simulink model "Controller_Observer_Model"  (R2021b)
settings: Solver=FixedStepAuto  StartTime=0.0  StopTime=10.0  RelTol=1e-3  EnableMultiTasking=on
undefined symbols (not defined in the file): Ad, Bd, Cd, DiscIntNeverNeededParam, ki, Kp, L, Ts
settings Model: ExtModeTrigDuration=10  Creator=UTENTE  LastModifiedBy=UTENTE
settings OptimizationCC: EnhancedBackFolding=on  PassReuseOutputArgsAs=Individual arguments  ZeroExternalMemoryAtStartup=off  ZeroInternalMemoryAtStartup=off  MaxStackSize=64  OptimizeBlockOrder=speed  DifferentSizesBufferReuse=on  OptimizationCustomize=off  EfficientTunableParamExpr=on
settings DebuggingCC: ParameterTunabilityLossMsg=error
settings HardwareCC: ProdBitPerPointer=32  ProdBitPerSizeT=32  ProdBitPerPtrDiffT=32  ProdLargestAtomicInteger=Long  ProdLargestAtomicFloat=Double  ProdWordSize=32  ProdLongLongMode=on  ProdHWDeviceType=ARM Compatible->ARM Cortex
settings SFSimCC: MATLABDynamicMemAlloc=off
settings RTWCC: Description=Embedded Coder  SystemTargetFile=ert.tlc  HardwareBoard=STM32 Nucleo F401RE  TemplateMakefile=ert_default_tmf  Toolchain=GNU Tools for ARM Embedded Processors  PortableWordSizes=on
settings CodeAppCC: ForceParamTrailComments=on  IgnoreCustomStorageClasses=off  OperatorAnnotations=on  SimulinkDataObjDesc=on  SFDataObjDesc=on  InsertBlockDesc=on
settings ERTTargetCC: ExtModeTransport=3  ExtModeStaticAlloc=on  ExtModeStaticAllocSize=2000  ExtModeMexFile=ext_xcp  ExtModeIntrfLevel=Level2 - Open

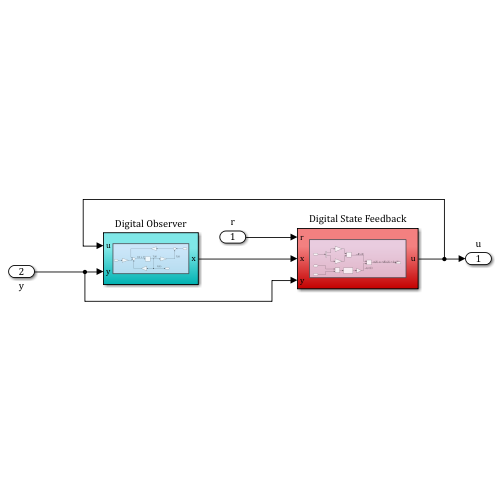
[thumbnail: Simulink's stored preview of the top-level diagram]
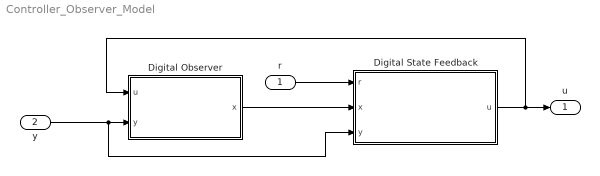
== system Controller_Observer_Model ==
  r : Inport
  y : Inport  Port=2
  Digital Observer : Subsystem
  Digital State Feedback : Subsystem
  u : Outport
  wires:
  r/1 -> Digital State Feedback/1(r)
  Digital State Feedback/1(u) -> Digital Observer/1(u), u/1
  Digital Observer/1(x) -> Digital State Feedback/2(x)
  y/1 -> Digital State Feedback/3(y), Digital Observer/2(y)

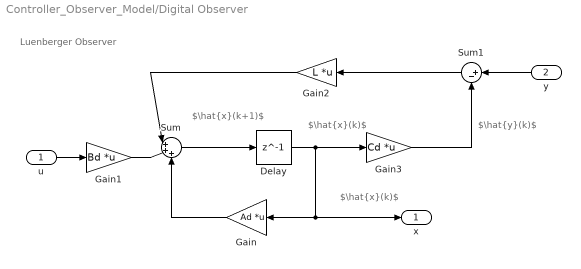
== system Controller_Observer_Model/Digital Observer ==
  note: $\hat{x}(k+1)$
  note: Luenberger Observer
  note: $\hat{x}(k)$
  note: $\hat{y}(k)$
  note: $\hat{x}(k)$
  u : Inport
  y : Inport  Port=2
  Delay : Delay  DelayLength=1  SampleTime=Ts
  Gain : Gain  Gain=Ad  Multiplication=Matrix(K*u)
  Gain1 : Gain  Gain=Bd  Multiplication=Matrix(K*u)
  Gain2 : Gain  Gain=L  Multiplication=Matrix(K*u)
  Gain3 : Gain  Gain=Cd  Multiplication=Matrix(K*u)
  Sum : Sum  Inputs=|+++
  Sum1 : Sum  Inputs=|+-
  x : Outport
  wires:
  u/1 -> Gain1/1
  Gain3/1 -> Sum1/2
  Delay/1 -> x/1, Gain/1, Gain3/1
  Gain1/1 -> Sum/2
  Gain2/1 -> Sum/1
  Sum/1 -> Delay/1
  Gain/1 -> Sum/3
  Sum1/1 -> Gain2/1
  y/1 -> Sum1/1

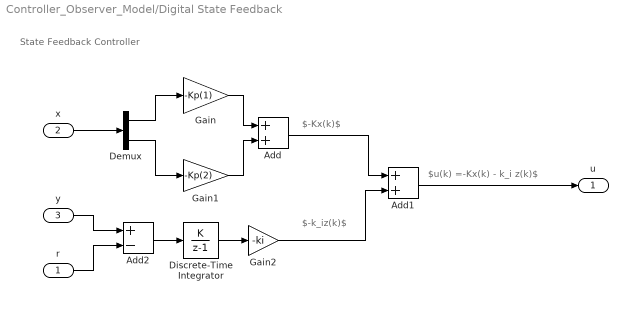
== system Controller_Observer_Model/Digital State Feedback ==
  note: $u(k) =-Kx(k) - k_i z(k)$
  note: $-k_iz(k)$
  note: $-Kx(k)$
  note: State Feedback Controller
  r : Inport
  x : Inport  Port=2
  y : Inport  Port=3
  Add : Sum
  Add1 : Sum
  Add2 : Sum  Inputs=+-
  Demux : Demux  Outputs=2
  Discrete-Time Integrator : DiscreteIntegrator  IntegratorMethod=Accumulation: Forward Euler  SampleTime=Ts  StateName='IntegralAction'  ICPrevOutput=DiscIntNeverNeededParam  ICPrevScaledInput=DiscIntNeverNeededParam
  Gain : Gain  Gain=-Kp(1)
  Gain1 : Gain  Gain=-Kp(2)
  Gain2 : Gain  Gain=-ki
  u : Outport
  wires:
  Gain/1 -> Add/1
  y/1 -> Add2/1
  Discrete-Time Integrator/1 -> Gain2/1
  Gain2/1 -> Add1/2
  x/1 -> Demux/1
  r/1 -> Add2/2
  Demux/2 -> Gain1/1
  Gain1/1 -> Add/2
  Add1/1 -> u/1
  Add/1 -> Add1/1
  Demux/1 -> Gain/1
  Add2/1 -> Discrete-Time Integrator/1
